simulink model "e7_1_1"  (R2018b)
settings: Solver=VariableStepAuto  StartTime=0.0  StopTime=10.0  RelTol=1e-3
values from neighbouring files (symbols this model uses):
  T = 0.2    [e7.m]
libraries: simulink x1
settings Model: Creator=hp  LastModifiedBy=hp

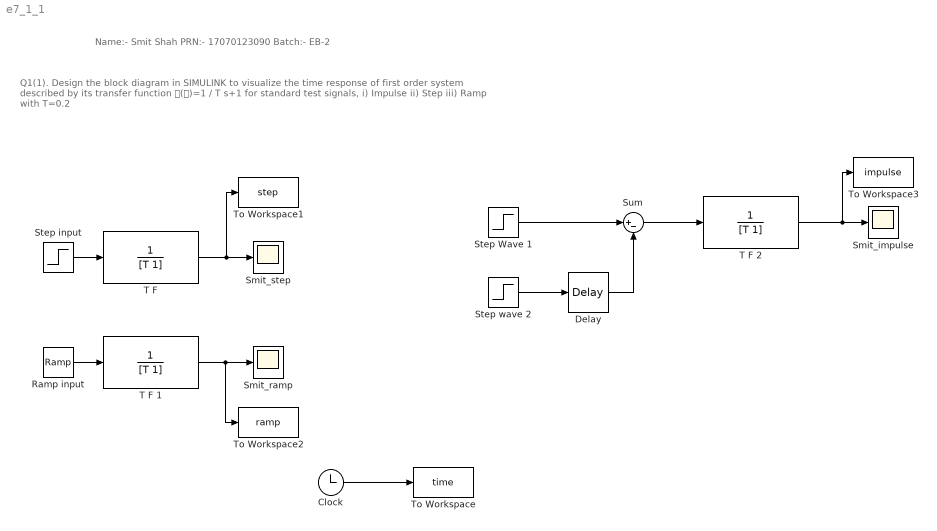
== system e7_1_1 ==
  note: Name:- Smit Shah PRN:- 17070123090 Batch:- EB-2
  note: Q1(1). Design the block diagram in SIMULINK to visualize the time response of first order system described by its
      | transfer function 𝐺(𝑠)=1 / T s+1 for standard test signals, i) Impulse ii) Step iii) Ramp with T=0.2
  Clock : Clock
  Delay : TransportDelay  DelayTime=0.00001
  Ramp input : simulink/Sources/Ramp  slope=1  start=0  InitialOutput=0
  Smit_impulse : Scope
  Smit_ramp : Scope
  Smit_step : Scope
  Step Wave 1 : Step  Time=0  SampleTime=0
  Step input : Step  SampleTime=0
  Step wave 2 : Step  Time=0  SampleTime=0
  Sum : Sum  Inputs=|+-
  T F : TransferFcn  Denominator=[T 1]
  T F 1 : TransferFcn  Denominator=[T 1]
  T F 2 : TransferFcn  Denominator=[T 1]
  To Workspace : ToWorkspace  VariableName=time  SampleTime=-1
  To Workspace1 : ToWorkspace  VariableName=step  SampleTime=-1
  To Workspace2 : ToWorkspace  VariableName=ramp  SampleTime=-1
  To Workspace3 : ToWorkspace  VariableName=impulse  SampleTime=-1
  wires:
  Delay/1 -> Sum/2
  Step wave 2/1 -> Delay/1
  Step Wave 1/1 -> Sum/1
  T F/1 -> To Workspace1/1, Smit_step/1
  Step input/1 -> T F/1
  T F 1/1 -> To Workspace2/1, Smit_ramp/1
  Ramp input/1 -> T F 1/1
  Sum/1 -> T F 2/1
  T F 2/1 -> To Workspace3/1, Smit_impulse/1
  Clock/1 -> To Workspace/1
